simulink model "Motor_Equation"  (R2022b)
settings: Solver=VariableStepAuto  StartTime=0.0  StopTime=10  RelTol=1e-3
model workspace (MAT data in the model file):
  J = 8.6
  Kd = 5
  Kf = 0.07
  Kg = 2000
  Kt = 0.07
  L = 1e-05
  R = 10
libraries: slpidlib x1
settings Model: Creator=adlercohen  LastModifiedBy=adlercohen
settings DataIOCC: ExternalInput=[sunTime, sunPosition]

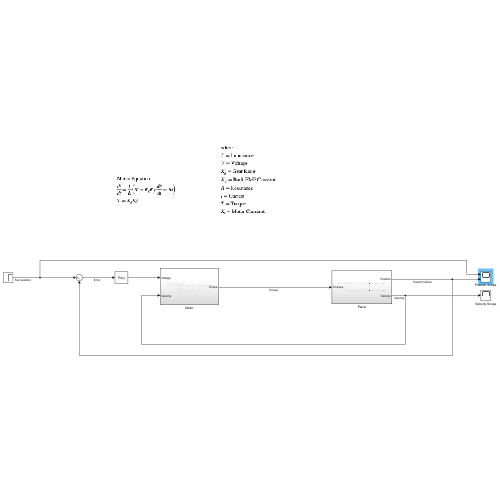
[thumbnail: Simulink's stored preview of the top-level diagram]
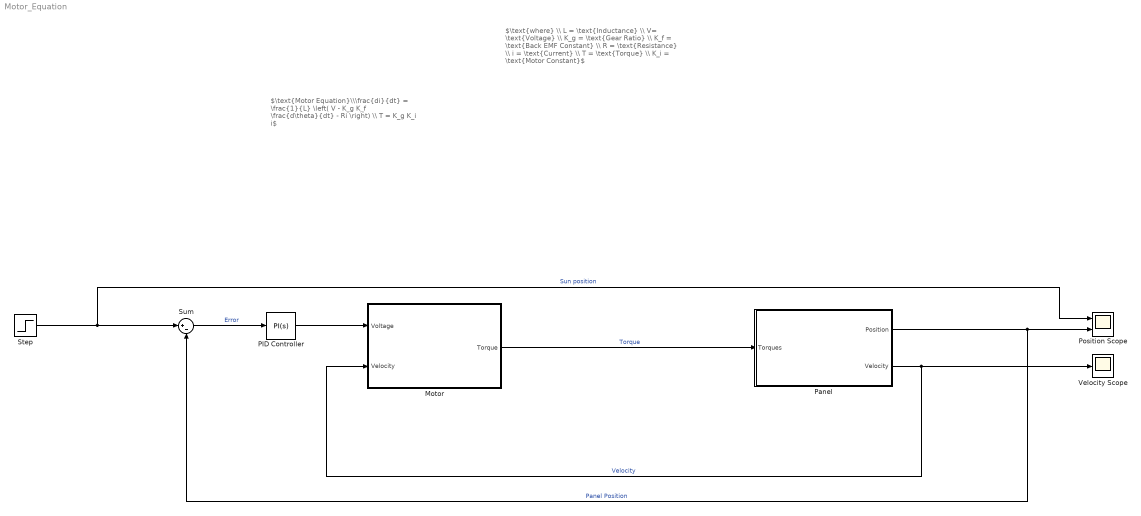
== system Motor_Equation ==
  note: $\text{where} \\ L = \text{Inductance} \\ V= \text{Voltage} \\ K_g = \text{Gear Ratio} \\ K_f = \text{Back EMF Constant} \\ R = \text{Resistance} \\ i = \text{Current} \\ T = \text{Torque} \\ K_i = \text{Motor Constant}$
  note: $\text{Motor Equation}\\\frac{di}{dt} = \frac{1}{L} \left( V - K_g K_f \frac{d\theta}{dt} - Ri \right) \\ T = K_g K_i i$
  Motor : Subsystem
  PID Controller : slpidlib/PID Controller  Controller=PI  Form=Parallel  TimeDomain=Continuous-time  UseExternalTs=off  SampleTime=-1  IntegratorMethod=Forward Euler  FilterMethod=Forward Euler  ControllerParametersSource=internal  P=240  I=180  UseKiTs=off  D=0  N=100  UseFilter=on  TunerSelectOption=Transfer Function Based (PID Tuner App)  InitialConditionSource=internal  InitialConditionForIntegrator=0  InitialConditionForFilter=0  DifferentiatorICPrevScaledInput=0  ExternalReset=none  TrackingMode=off  Kt=1  LimitOutput=off  SatLimitsSource=internal  UpperSaturationLimit=inf  LowerSaturationLimit=-inf  LinearizeAsGain=on  AntiWindupMode=none  Kb=1  LimitIntegrator=off  UpperIntegratorSaturationLimit=inf  LowerIntegratorSaturationLimit=-inf  POutMin=[]  POutMax=[]  IOutMin=[]  IOutMax=[]  DOutMin=[]  DOutMax=[]  NOutMin=[]  NOutMax=[]  SumOutMin=[]  SumOutMax=[]  SaturationOutMin=[]  SaturationOutMax=[]  PParamMin=[]  PParamMax=[]  IParamMin=[]  IParamMax=[]  DParamMin=[]  DParamMax=[]  NParamMin=[]  NParamMax=[]  KbParamMin=[]  KbParamMax=[]  KtParamMin=[]  KtParamMax=[]  KbOutMin=[]  KbOutMax=[]  KtOutMin=[]  KtOutMax=[]  IntegratorOutMin=[]  IntegratorOutMax=[]  FilterOutMin=[]  FilterOutMax=[]  SumI1OutMin=[]  SumI1OutMax=[]  SumI2OutMin=[]  SumI2OutMax=[]  SumI3OutMin=[]  SumI3OutMax=[]  SumI4OutMin=[]  SumI4OutMax=[]  SumDOutMin=[]  SumDOutMax=[]  DifferentiatorOutMin=[]  DifferentiatorOutMax=[]  FilterDiffOutCoefMin=[]  FilterDiffOutCoefMax=[]  ReciprocalOutMin=[]  ReciprocalOutMax=[]  SumDenOutMin=[]  SumDenOutMax=[]  SumNumOutMin=[]  SumNumOutMax=[]  DivideOutMin=[]  DivideOutMax=[]  UdiffTsProdOutMin=[]  UdiffTsProdOutMax=[]  NTsProdOutMin=[]  NTsProdOutMax=[]  UintegralTsProdOutMin=[]  UintegralTsProdOutMax=[]  UngainTsProdOutMin=[]  UngainTsProdOutMax=[]  ClampingZeroOutDataTypeStr=Inherit: Inherit via back propagation  ClampingZeroOutMin=[]  ClampingZeroOutMax=[]  FilterDenConstantOutDataTypeStr=Inherit: Inherit via back propagation  FilterDenConstantOutMin=[]  FilterDenConstantOutMax=[]  PCopyOutDataTypeStr=Inherit: Inherit via back propagation  PCopyOutMin=[]  PCopyOutMax=[]  NCopyOutDataTypeStr=Inherit: Inherit via back propagation  NCopyOutMin=[]  NCopyOutMax=[]  IntegratorContinuousStateAttributes=''  IntegratorStateMustResolveToSignalObject=off  IntegratorRTWStateStorageClass=Auto  FilterContinuousStateAttributes=''  FilterStateMustResolveToSignalObject=off  FilterRTWStateStorageClass=Auto  ParallelPVariant=InternalParameters  IdealPVariant=Disabled  IVariant=InternalParameters  DVariant=Disabled  IntegratorVariant=Continuous  SatVariant=Disabled  AWVariant=Passthrough  PCopyVariant=Disabled  TRVariant=Disabled  FdbkBlocksVariant=Forward  IdealPFdbkVariant=Disabled  SatFdbkVariant=Disabled  DerivativeFilterVariant=Disabled  NVariant=Disabled  NCopyVariant=Disabled_SignalSpec  FilterICVariant=Disabled  IntegratorICVariant=InternalICs  ExternalResetVariant=Disabled  TRSumVariant=Passthrough  SumFdbkVariant=Disabled  SumVariant=Sum_PI  TsampFilterVariant=InternalTs  TsampNgainVariant=Passthrough  TsampIntegralVariant=Passthrough  ExternalSaturationOutDataTypeStr=Inherit: Same as second input
  Panel : Subsystem
  Position Scope : Scope  NumInputPorts=2
  Step : Step  SampleTime=0
  Sum : Sum  Inputs=|+-
  Velocity Scope : Scope
  wires:
  Panel/2(Velocity) -> Velocity Scope/1, Motor/2(Velocity)  "Velocity"
  Panel/1(Position) -> Sum/2, Position Scope/2  "Panel Position"
  Motor/1(Torque) -> Panel/1(Torques)  "Torque"
  Step/1 -> Position Scope/1, Sum/1  "Sun position"
  Sum/1 -> PID Controller/1  "Error"
  PID Controller/1 -> Motor/1(Voltage)

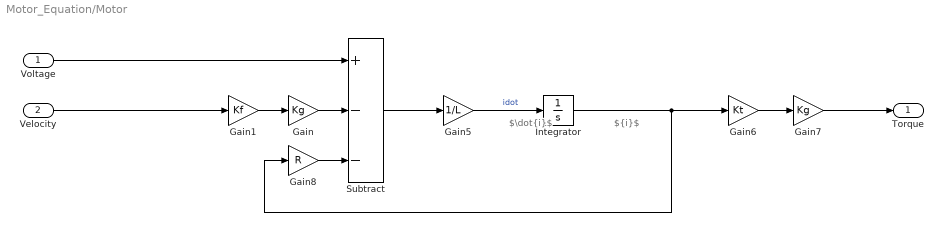
== system Motor_Equation/Motor ==
  note: $\dot{i}$
  note: ${i}$
  Voltage : Inport
  Velocity : Inport  Port=2
  Gain : Gain  Gain=Kg
  Gain1 : Gain  Gain=Kf
  Gain5 : Gain  Gain=1/L
  Gain6 : Gain  Gain=Kt
  Gain7 : Gain  Gain=Kg
  Gain8 : Gain  Gain=R
  Integrator : Integrator
  Subtract : Sum  Inputs=+--
  Torque : Outport
  wires:
  Gain/1 -> Subtract/2
  Subtract/1 -> Gain5/1
  Gain8/1 -> Subtract/3
  Integrator/1 -> Gain8/1, Gain6/1
  Gain6/1 -> Gain7/1
  Gain5/1 -> Integrator/1  "idot"
  Gain1/1 -> Gain/1
  Gain7/1 -> Torque/1
  Voltage/1 -> Subtract/1
  Velocity/1 -> Gain1/1

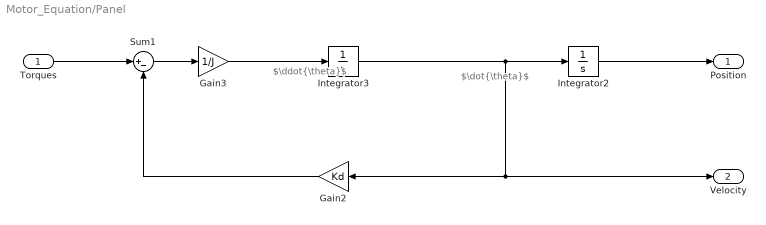
== system Motor_Equation/Panel ==
  note: $\ddot{\theta}$
  note: $\dot{\theta}$
  Torques : Inport
  Gain2 : Gain  Gain=Kd
  Gain3 : Gain  Gain=1/J
  Integrator2 : Integrator
  Integrator3 : Integrator
  Sum1 : Sum  Inputs=|+-
  Position : Outport
  Velocity : Outport  Port=2
  wires:
  Torques/1 -> Sum1/1
  Integrator3/1 -> Velocity/1, Gain2/1, Integrator2/1
  Gain2/1 -> Sum1/2
  Sum1/1 -> Gain3/1
  Integrator2/1 -> Position/1
  Gain3/1 -> Integrator3/1
